simulink library "dspparest2"  (Simulink 3.00)
libraries: dspmtrx2 x14, dspvect2 x4, dsplinalg x3, simulink3 x3, dspelem2 x2, dspbdsp2 x1
settings Model: Creator=don  LastModifiedBy=don

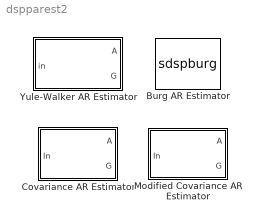
== system dspparest2 ==
  Burg AR Estimator : S-Function  FunctionName=sdspburg  Parameters=ord,fcn  PortCounts=[]  SFunctionModules=''  mask(Burg AR Estimator){fcn=A, ord=4}
      mask prompts: fcn "Output(s):"; ord "Order:"
      mask help: Frame-based parametric AR estimation using the Burg maximum entropy method. Outputs AR model coefficients A and/or reflection coefficients K, plus the model gain, G.
      mask init:
      | s = dspblkburg(fcn);
      mask Help: web(dspbhelp);
      mask StyleString: popup(A and K|A|K),edit
      mask Display:
      | disp('Burg AR\nEstimator');
      | port_label('output',s.o1,s.o1s);
      | port_label('output',s.o2,s.o2s);
      | port_label('output',s.o3,s.o3s);
  Covariance AR Estimator : Subsystem  mask(Covariance AR Estimator){bufsiz=10, ord=4}
      mask prompts: bufsiz "Input frame size:"; ord "Order:"
      mask help: Frame-based parametric AR estimation using the Covariance method. The AR model coefficients are given in A and the gain is given in G.
      mask Help: web(dspbhelp);
      mask Display: disp('Cov AR\nEstimator')
  Modified Covariance AR Estimator : Subsystem  mask(Modified Covariance AR Estimator){bufsiz=10, ord=4}
      mask prompts: bufsiz "Input frame size:"; ord "Order:"
      mask help: Frame-based parametric AR estimation using the Modified Covariance method. The AR model coefficients are given in A and the gain is given in G.
      mask Help: web(dspbhelp);
      mask Display: disp('MCov AR\nEstimator')
  Yule-Walker AR Estimator : Subsystem  mask(Yule-Walker AR Estimator){ord=-1}
      mask prompts: ord "Order (-1 for length(u)-1):"
      mask help: Frame-based parametric AR estimation using the Yule-Walker method. The AR model coefficients are given in A and the gain is given in G.
      mask init:
      | if ord==-1,
      |    pad = -1; acf=-1;
      | else
      |    pad = ord+1; acf=ord;
      | end
      mask Help: web(dspbhelp);
      mask Display: disp('Yule AR\nEstimator')

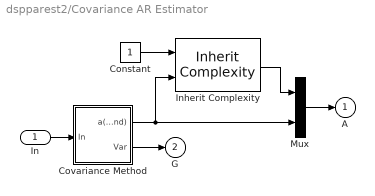
== system dspparest2/Covariance AR Estimator ==
  In : Inport  Port=1  PortWidth=-1  SampleTime=-1  DataType=auto
      settings: SignalType=auto
  Constant : Constant  Value=1
  Covariance Method : Subsystem
  Inherit Complexity : dspelem2/Inherit Complexity
  Mux : Mux  Inputs=2
  A : Outport  Port=1  InitialOutput=0
  G : Outport  Port=2  InitialOutput=0
  wires:
  In/1 -> Covariance Method/1(In)
  Mux/1 -> A/1
  Covariance Method/1(a(2:end)) -> Mux/2, Inherit Complexity/2
  Constant/1 -> Inherit Complexity/1
  Inherit Complexity/1 -> Mux/1
  Covariance Method/2(Var) -> G/1

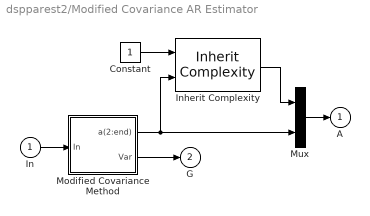
== system dspparest2/Modified Covariance AR Estimator ==
  In : Inport  Port=1  PortWidth=-1  SampleTime=-1  DataType=auto
      settings: SignalType=auto
  Constant : Constant  Value=1
  Inherit Complexity : dspelem2/Inherit Complexity
  Modified Covariance Method : Subsystem
  Mux : Mux  Inputs=2
  A : Outport  Port=1  InitialOutput=0
  G : Outport  Port=2  InitialOutput=0
  wires:
  Mux/1 -> A/1
  Modified Covariance Method/1(a(2:end)) -> Mux/2, Inherit Complexity/2
  Constant/1 -> Inherit Complexity/1
  Inherit Complexity/1 -> Mux/1
  Modified Covariance Method/2(Var) -> G/1
  In/1 -> Modified Covariance Method/1(In)

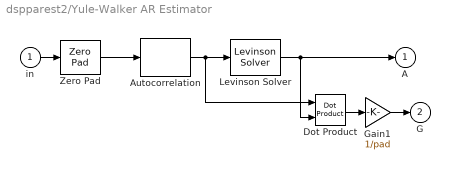
== system dspparest2/Yule-Walker AR Estimator ==
  in : Inport  Port=1  PortWidth=-1  SampleTime=-1  DataType=auto
      settings: SignalType=auto
  Autocorrelation : dspvect2/Autocorrelation  maxlag=acf  bias=Biased
  Dot Product : simulink3/Math/Dot Product
  Gain1 : Gain  Gain=1/pad  SaturateOnIntegerOverflow=on
  Levinson Solver : dsplinalg/Levinson Solver  fcn=A  otype=on
  Zero Pad : dspbdsp2/Zero Pad  pad=pad  trunc=off  nchans=1
  A : Outport  Port=1  InitialOutput=0
  G : Outport  Port=2  InitialOutput=0
  wires:
  in/1 -> Zero Pad/1
  Autocorrelation/1 -> Levinson Solver/1, Dot Product/1
  Levinson Solver/1 -> A/1, Dot Product/2
  Zero Pad/1 -> Autocorrelation/1
  Dot Product/1 -> Gain1/1
  Gain1/1 -> G/1

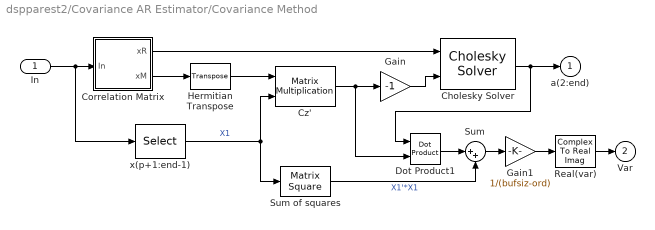
== system dspparest2/Covariance AR Estimator/Covariance Method ==
  In : Inport  Port=1  PortWidth=-1  SampleTime=-1  DataType=auto
      settings: SignalType=auto
  Cholesky Solver : dsplinalg/Cholesky Solver  errmode=Warning
  Correlation Matrix : Subsystem
  Cz' : dspmtrx2/Matrix Multiplication  Asize=[ord bufsiz-ord]  Bcols=1
  Dot Product1 : simulink3/Math/Dot Product
  Gain : Gain  Gain=-1  SaturateOnIntegerOverflow=on
  Gain1 : Gain  Gain=1/(bufsiz-ord)  SaturateOnIntegerOverflow=on
  Hermitian Transpose : dspmtrx2/Transpose  Asize=ord  Hermitian=on
  Real(var) : ComplexToRealImag  Output=Real
  Sum : Sum  Inputs=|++  SaturateOnIntegerOverflow=on
  Sum of squares : dspmtrx2/Matrix Square  Acols=1
  x(p+1:end-1) : Selector  Elements=ord+1:bufsiz  InputPortWidth=bufsiz
  a(2:end) : Outport  Port=1  InitialOutput=0
  Var : Outport  Port=2  InitialOutput=0
  wires:
  In/1 -> x(p+1:end-1)/1, Correlation Matrix/1(In)
  Cz'/1 -> Dot Product1/2, Gain/1
  x(p+1:end-1)/1 -> Cz'/2, Sum of squares/1  "X1"
  Correlation Matrix/2(xM) -> Hermitian Transpose/1
  Hermitian Transpose/1 -> Cz'/1
  Gain/1 -> Cholesky Solver/2
  Correlation Matrix/1(xR) -> Cholesky Solver/1
  Cholesky Solver/1 -> Dot Product1/1, a(2:end)/1
  Sum/1 -> Gain1/1
  Dot Product1/1 -> Sum/1
  Real(var)/1 -> Var/1
  Gain1/1 -> Real(var)/1
  Sum of squares/1 -> Sum/2  "X1'*X1"

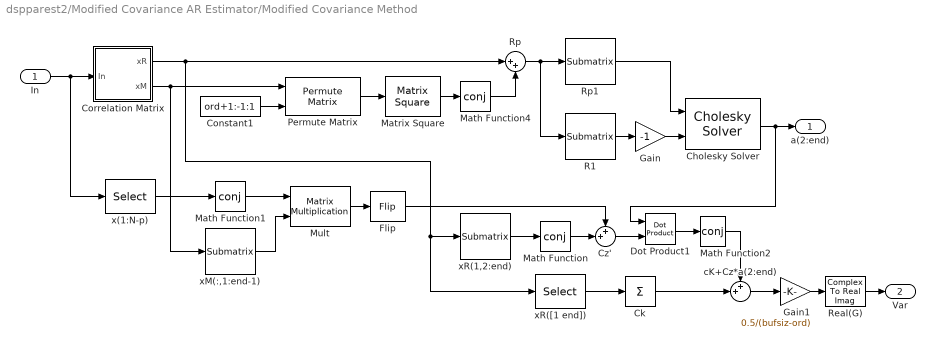
== system dspparest2/Modified Covariance AR Estimator/Modified Covariance Method ==
  In : Inport  Port=1  PortWidth=-1  SampleTime=-1  DataType=auto
      settings: SignalType=auto
  Cholesky Solver : dsplinalg/Cholesky Solver  errmode=Warning
  Ck : Sum  Inputs=1  SaturateOnIntegerOverflow=on
  Constant1 : Constant  Value=ord+1:-1:1
  Correlation Matrix : Subsystem
  Cz' : Sum  Inputs=++|  SaturateOnIntegerOverflow=on
  Dot Product1 : simulink3/Math/Dot Product
  Flip : dspvect2/Flip
  Gain : Gain  Gain=-1  SaturateOnIntegerOverflow=on
  Gain1 : Gain  Gain=0.5/(bufsiz-ord)  SaturateOnIntegerOverflow=on
  Math Function{,1..2,4} (4 alike) : Math  Operator=conj  OutputSignalType=auto
  Matrix Square : dspmtrx2/Matrix Square  Acols=ord+1
  Mult : dspmtrx2/Matrix Multiplication  Asize=[1 bufsiz-ord]  Bcols=ord
  Permute Matrix : dspmtrx2/Permute Matrix  mode=Columns  errmode=Clip Index  cols=ord+1
  R1 : dspmtrx2/Submatrix  siz=[ord+1 ord+1]  expr={2:ord+1,1}
  Real(G) : ComplexToRealImag  Output=Real
  Rp : Sum  Inputs=|++  SaturateOnIntegerOverflow=on
  Rp1 : dspmtrx2/Submatrix  siz=[ord+1 ord+1]  expr={2:ord+1, 2:ord+1}
  cK+Cz*a(2:end) : Sum  Inputs=++|  SaturateOnIntegerOverflow=on
  x(1:N-p) : Selector  Elements=1:bufsiz-ord  InputPortWidth=bufsiz
  xM(:,1:end-1) : dspmtrx2/Submatrix  siz=[bufsiz-ord ord+1]  expr={1:bufsiz-ord, 1:ord}
  xR(1,2:end) : dspmtrx2/Submatrix  siz=[ord+1 ord+1]  expr={1, 2:ord+1}
  xR([1 end]) : Selector  Elements=[1 (ord+1)*(ord+1)]  InputPortWidth=(ord+1)*(ord+1)
  a(2:end) : Outport  Port=1
  Var : Outport  Port=2
  wires:
  Cholesky Solver/1 -> a(2:end)/1, Dot Product1/1
  Rp/1 -> R1/1, Rp1/1
  R1/1 -> Gain/1
  Gain/1 -> Cholesky Solver/2
  Rp1/1 -> Cholesky Solver/1
  Correlation Matrix/1(xR) -> xR(1,2:end)/1, xR([1 end])/1, Rp/1
  Correlation Matrix/2(xM) -> Permute Matrix/1, xM(:,1:end-1)/1
  In/1 -> x(1:N-p)/1, Correlation Matrix/1(In)
  Constant1/1 -> Permute Matrix/2
  Math Function4/1 -> Rp/2
  Permute Matrix/1 -> Matrix Square/1
  Matrix Square/1 -> Math Function4/1
  xM(:,1:end-1)/1 -> Mult/2
  Math Function1/1 -> Mult/1
  x(1:N-p)/1 -> Math Function1/1
  xR([1 end])/1 -> Ck/1
  Math Function/1 -> Cz'/2
  xR(1,2:end)/1 -> Math Function/1
  Flip/1 -> Cz'/1
  Mult/1 -> Flip/1
  Dot Product1/1 -> Math Function2/1
  Cz'/1 -> Dot Product1/2
  Gain1/1 -> Real(G)/1
  cK+Cz*a(2:end)/1 -> Gain1/1
  Ck/1 -> cK+Cz*a(2:end)/2
  Real(G)/1 -> Var/1
  Math Function2/1 -> cK+Cz*a(2:end)/1

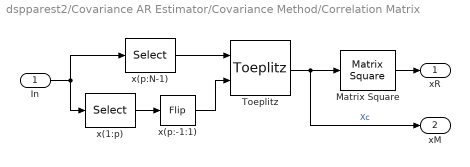
== system dspparest2/Covariance AR Estimator/Covariance Method/Correlation Matrix ==
  In : Inport  Port=1  PortWidth=-1  SampleTime=-1  DataType=auto
      settings: SignalType=auto
  Matrix Square : dspmtrx2/Matrix Square  Acols=ord
  Toeplitz : dspmtrx2/Toeplitz  Symmetric=off
  x(1:p) : Selector  Elements=1:ord  InputPortWidth=bufsiz
  x(p:-1:1) : dspvect2/Flip
  x(p:N-1) : Selector  Elements=ord:bufsiz-1  InputPortWidth=bufsiz
  xR : Outport  Port=1
  xM : Outport  Port=2
  wires:
  x(1:p)/1 -> x(p:-1:1)/1
  x(p:N-1)/1 -> Toeplitz/1
  x(p:-1:1)/1 -> Toeplitz/2
  Toeplitz/1 -> Matrix Square/1, xM/1  "Xc"
  In/1 -> x(p:N-1)/1, x(1:p)/1
  Matrix Square/1 -> xR/1

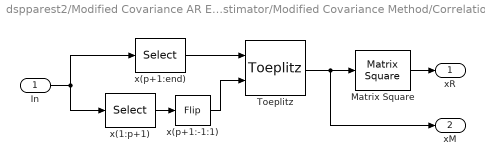
== system dspparest2/Modified Covariance AR Estimator/Modified Covariance Method/Correlation Matrix ==
  In : Inport  Port=1  PortWidth=-1  SampleTime=-1  DataType=auto
      settings: SignalType=auto
  Matrix Square : dspmtrx2/Matrix Square  Acols=ord+1
  Toeplitz : dspmtrx2/Toeplitz  Symmetric=off
  x(1:p+1) : Selector  Elements=1:ord+1  InputPortWidth=bufsiz
  x(p+1:-1:1) : dspvect2/Flip
  x(p+1:end) : Selector  Elements=ord+1:bufsiz  InputPortWidth=bufsiz
  xR : Outport  Port=1
  xM : Outport  Port=2
  wires:
  x(1:p+1)/1 -> x(p+1:-1:1)/1
  Toeplitz/1 -> Matrix Square/1, xM/1
  In/1 -> x(1:p+1)/1, x(p+1:end)/1
  x(p+1:-1:1)/1 -> Toeplitz/2
  x(p+1:end)/1 -> Toeplitz/1
  Matrix Square/1 -> xR/1
